simulink model "Lcontainer_simNN"  (R2018b)
settings: Solver=FixedStepAuto  StartTime=0.0  StopTime=50  FixedStep=0.1  RelTol=1e-3
libraries: neural x548, simulink x2
(part 9 of 26)

== system Lcontainer_simNN/Lcontainer Plant/NN Plant LContainer/Layer 5/Delays 1 ==
  "p{5}" : Inport  PortDimensions=30
      mask Display: e = 0.06;c1 = [120 230 180]/255;c2 = ([120 230 180]+0)/(256+128);c3 = ([120 230 180]+128)/(256+128);patch([0 1 1 0],[0 0 1 1],c1);patch([0 1 1 1-e 1-e 0+e],[0 0 1 1-e 0+e 0+e],c2);patch([0 0 1 1-e 0+e 0+e],[0 1 1 1-e 1-e 0+e],c3);plot([0 1 1 0 0],[0 0 1 1 0]);
  mux : Mux  Inputs=1
      mask Display: e = 0.06;c1 = [120 150 230]/255;c2 = ([120 150 230]+0)/383;c3 = ([120 150 230]+128)/383;patch([0 1 1 0],[0 0 1 1],c1);patch([0 1 1 1-e 1-e 0+e],[0 0 1 1-e 0+e 0+e],c2);patch([0 0 1 1-e 0+e 0+e],[0 1 1 1-e 1-e 0+e],c3);plot([0 1 1 0 0],[0 0 1 1 0]);disp('Mux')
  "pd{5,4}" : Outport
      mask Display: e = 0.06;c1 = [120 230 180]/255;c2 = ([120 230 180]+0)/(256+128);c3 = ([120 230 180]+128)/(256+128);patch([0 1 1 0],[0 0 1 1],c1);patch([0 1 1 1-e 1-e 0+e],[0 0 1 1-e 0+e 0+e],c2);patch([0 0 1 1-e 0+e 0+e],[0 1 1 1-e 1-e 0+e],c3);plot([0 1 1 0 0],[0 0 1 1 0]);
  wires:
  mux/1 -> "pd{5,4}"/1
  "p{5}"/1 -> mux/1

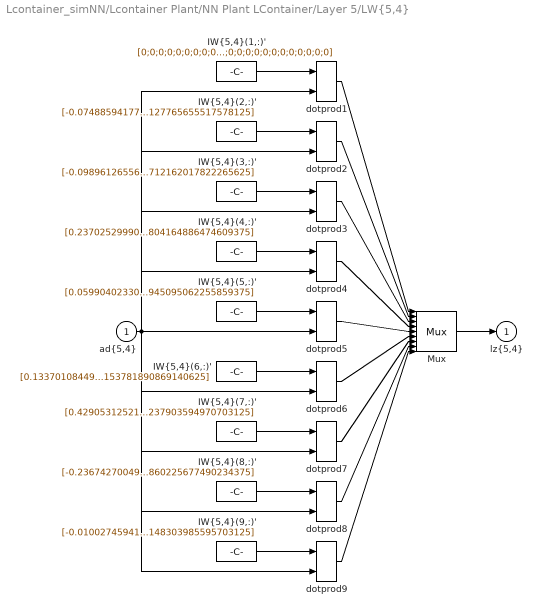
== system Lcontainer_simNN/Lcontainer Plant/NN Plant LContainer/Layer 5/LW{5,4} ==
  "ad{5,4}" : Inport  PortDimensions=30
      mask Display: e = 0.06;c1 = [120 230 180]/255;c2 = ([120 230 180]+0)/(256+128);c3 = ([120 230 180]+128)/(256+128);patch([0 1 1 0],[0 0 1 1],c1);patch([0 1 1 1-e 1-e 0+e],[0 0 1 1-e 0+e 0+e],c2);patch([0 0 1 1-e 0+e 0+e],[0 1 1 1-e 1-e 0+e],c3);plot([0 1 1 0 0],[0 0 1 1 0]);
  "IW{5,4}(1,:)'" : Constant  Value=[0;0;0;0;0;0;0;0;0;0;0;0;0;0;0;0;0;0;0;0;0;0;0;0;0;0;0;0;0;0]
      mask Display: e = 0.06;c1 = [120 150 230]/255;c2 = ([120 150 230]+0)/383;c3 = ([120 150 230]+128)/383;patch([0 1 1 0],[0 0 1 1],c1);patch([0 1 1 1-e 1-e 0+e],[0 0 1 1-e 0+e 0+e],c2);patch([0 0 1 1-e 0+e 0+e],[0 1 1 1-e 1-e 0+e],c3);plot([0 1 1 0 0],[0 0 1 1 0]);disp('weights');
  "IW{5,4}(2,:)'" : Constant  Value=[-0.0748859417790649073420894410446635447442531585693359375;-0.04828556424962082704865906634950079023838043212890625;-0.033114210472323622747037319413720979355275630950927734375;0;-0.1705933706616073741724193268964882008731365203857421875;-0.024529633517243805418406310536738601513206958770751953125;0.0021195137212356375717992040819126486894674599170684814453125;0.01236919402911206000705846008713706396520137786865234375;0;0.14372941073911327247714098120923154056072235107421875;-0.08898138145787300168354505558454548008739948272705078125;0.25399576565349579748698261028039269149303436279296875;0;0;0.0852243252470792078678840653083170764148235321044921875;-0.01075542795457371143819091940940779750235378742218017578125;-0.445323566962354366882692602302995510399341583251953125;0;0;-0.09295428806737338067733844582107849419116973876953125;0;0.01344213504127246376629312152317652362398803234100341796875;0.032260333898478661673880907301281695254147052764892578125;0;0.09247761640926364934411907370304106734693050384521484375;0;-0.168932518774683571027850348400534130632877349853515625;0.0852925813085265438484583455647225491702556610107421875;0;0.06589481023012284943707328466189210303127765655517578125]
      mask Display: e = 0.06;c1 = [120 150 230]/255;c2 = ([120 150 230]+0)/383;c3 = ([120 150 230]+128)/383;patch([0 1 1 0],[0 0 1 1],c1);patch([0 1 1 1-e 1-e 0+e],[0 0 1 1-e 0+e 0+e],c2);patch([0 0 1 1-e 0+e 0+e],[0 1 1 1-e 1-e 0+e],c3);plot([0 1 1 0 0],[0 0 1 1 0]);disp('weights');
  "IW{5,4}(3,:)'" : Constant  Value=[-0.09896126556202029800335395748334121890366077423095703125;0.0796723090629556096597951864168862812221050262451171875;-0.0127063350048920893631265727208301541395485401153564453125;0;0.057556295472263131751677889269558363594114780426025390625;0.2154824786930362723325060869683511555194854736328125;0.000775384221512636306015975318217670064768753945827484130859375;0.0271174472186132727025142941101876203902065753936767578125;0;-0.371698716803673889774728422707994468510150909423828125;-0.146328714086319866538588030380196869373321533203125;0.0713073127667704642629331601710873655974864959716796875;0;0;-0.2355891362308875913722516770576476119458675384521484375;-0.30076611836778355257848716064472682774066925048828125;-0.1185366313755974732035980423461296595633029937744140625;0;0;0.1996103508031047690796100368970655836164951324462890625;0;0.05914976055061747783891945573486736975610256195068359375;0.0178303994357455440622484132973113446496427059173583984375;0;0.1153034810071617843885150023197638802230358123779296875;0;-0.045867220948066007857324422047895495779812335968017578125;0.259149319149599433043107410412630997598171234130859375;0;0.03300873027772155410275445319712162017822265625]
      mask Display: e = 0.06;c1 = [120 150 230]/255;c2 = ([120 150 230]+0)/383;c3 = ([120 150 230]+128)/383;patch([0 1 1 0],[0 0 1 1],c1);patch([0 1 1 1-e 1-e 0+e],[0 0 1 1-e 0+e 0+e],c2);patch([0 0 1 1-e 0+e 0+e],[0 1 1 1-e 1-e 0+e],c3);plot([0 1 1 0 0],[0 0 1 1 0]);disp('weights');
  "IW{5,4}(4,:)'" : Constant  Value=[0.237025299903385555655432881394517607986927032470703125;-0.09628402043828758471999407220209832303225994110107421875;0.1610493651533241032947074700132361613214015960693359375;0;0.1525638746941407053459016651686397381126880645751953125;-0.369699757752953439560172910205437801778316497802734375;0.04575628933936337627841339781298302114009857177734375;-0.0272463917095127523826381121807571616955101490020751953125;0;0.1707957341201938039620955578357097692787647247314453125;0.1980833692316685823442412583972327411174774169921875;0.34262854725739433359166241643833927810192108154296875;0;0;-0.440432226404521121043700304653611965477466583251953125;-0.0306731198290640764969605669421071070246398448944091796875;-0.11361114234840441472584871007711626589298248291015625;0;0;0.161134980998437982169235738183488138020038604736328125;0;-0.1919326921231571392301162859439500607550144195556640625;-0.18954446100379473971742072535562328994274139404296875;0;0.10598471434648359945640549995005130767822265625;0;0.09503752363470081843122017062341910786926746368408203125;0.1143533842217742402258551237537176348268985748291015625;0;-0.6652481266117751257382906260318122804164886474609375]
      mask Display: e = 0.06;c1 = [120 150 230]/255;c2 = ([120 150 230]+0)/383;c3 = ([120 150 230]+128)/383;patch([0 1 1 0],[0 0 1 1],c1);patch([0 1 1 1-e 1-e 0+e],[0 0 1 1-e 0+e 0+e],c2);patch([0 0 1 1-e 0+e 0+e],[0 1 1 1-e 1-e 0+e],c3);plot([0 1 1 0 0],[0 0 1 1 0]);disp('weights');
  "IW{5,4}(5,:)'" : Constant  Value=[0.05990402330856892110233502535265870392322540283203125;0.00141316250715774042491512663133335081511177122592926025390625;-0.2434454959196580003943921610698453150689601898193359375;0;0.0717643993970850380126336176545009948313236236572265625;0.028162462427314925716981264258720329962670803070068359375;0.0094946210627239562007684270383833791129291057586669921875;-0.055190171920815551953598543377665919251739978790283203125;0;-0.0250218219302644727386475409502963884733617305755615234375;0.012124972570229854140766434511533589102327823638916015625;0.13711765032037870337688900690409354865550994873046875;0;0;0.09628367634003372199646975104769808240234851837158203125;-0.00681706128747262829481456947178230620920658111572265625;0.1430879199190295825161456377827562391757965087890625;0;0;0.0239743569962188492195043210131188970990478992462158203125;0;-0.08149740200468764961261314283547108061611652374267578125;0.010347551788515589599182220581496949307620525360107421875;0;0.05234499219716891305065331607693224214017391204833984375;0;0.0880266504674781236072789170066243968904018402099609375;-0.00576249198361480398367096000811216072179377079010009765625;0;0.056000545253366527942429087261189124546945095062255859375]
      mask Display: e = 0.06;c1 = [120 150 230]/255;c2 = ([120 150 230]+0)/383;c3 = ([120 150 230]+128)/383;patch([0 1 1 0],[0 0 1 1],c1);patch([0 1 1 1-e 1-e 0+e],[0 0 1 1-e 0+e 0+e],c2);patch([0 0 1 1-e 0+e 0+e],[0 1 1 1-e 1-e 0+e],c3);plot([0 1 1 0 0],[0 0 1 1 0]);disp('weights');
  "IW{5,4}(6,:)'" : Constant  Value=[0.133701084498613287365742507972754538059234619140625;-0.08509330829521111194679861000622622668743133544921875;-0.0205939214417339526430605900486625614576041698455810546875;0;0.17660601722820679082559536254848353564739227294921875;-0.0985909020102693489651102254356374032795429229736328125;-0.006612346173665164562882612386829350725747644901275634765625;0.035407645810061887103881161920071463100612163543701171875;0;0.12139874970078590177280375428381375968456268310546875;-0.04879072530735041601790413778871879912912845611572265625;0.046767611231733612064953575782055850140750408172607421875;0;0;0.07297241468848725265416987895150668919086456298828125;0.029678867821005351645968772800188162364065647125244140625;0.11596813525751230311566786213006707839667797088623046875;0;0;0.029034809825560538298905299825491965748369693756103515625;0;0.07527837444470493466486260558667709119617938995361328125;-0.02440627391344178664933650679813581518828868865966796875;0;0.138042976115350046750762658120947889983654022216796875;0;-0.07122006785791994143419714191622915677726268768310546875;-0.1535383105928499192227576486402540467679500579833984375;0;0.07388509161200375319200617241222062148153781890869140625]
      mask Display: e = 0.06;c1 = [120 150 230]/255;c2 = ([120 150 230]+0)/383;c3 = ([120 150 230]+128)/383;patch([0 1 1 0],[0 0 1 1],c1);patch([0 1 1 1-e 1-e 0+e],[0 0 1 1-e 0+e 0+e],c2);patch([0 0 1 1-e 0+e 0+e],[0 1 1 1-e 1-e 0+e],c3);plot([0 1 1 0 0],[0 0 1 1 0]);disp('weights');
  "IW{5,4}(7,:)'" : Constant  Value=[0.42905312521970484507249921080074273049831390380859375;0.1906589972924225551142995982445427216589450836181640625;-0.2203038801554847714303519978784606792032718658447265625;0;0.0217157024741243230570031386150731123052537441253662109375;0.00986713763709344722496741297845801454968750476837158203125;-0.0015074870746090672513073371874270378611981868743896484375;-0.00103538587713326683814596407273711520247161388397216796875;0;-0.334719609204135737368090985910384915769100189208984375;-0.321965949665375450461368700416642241179943084716796875;0.030844820817152888980938740814963239245116710662841796875;0;0;0.01779259507096221659683266125284717418253421783447265625;0.3773025667999700960564268825692124664783477783203125;-0.12169499692181691419268219078730908222496509552001953125;0;0;-0.352967196418212225683674887477536685764789581298828125;0;0.37503733804256977890645430306904017925262451171875;-0.0031221649642524753644201584990014453069306910037994384765625;0;-0.12199386878124203470452613373709027655422687530517578125;0;-0.0686099962025387422048794405782246030867099761962890625;0.2458374314142147409878447206210694275796413421630859375;0;-0.262765638305728910228964423367870040237903594970703125]
      mask Display: e = 0.06;c1 = [120 150 230]/255;c2 = ([120 150 230]+0)/383;c3 = ([120 150 230]+128)/383;patch([0 1 1 0],[0 0 1 1],c1);patch([0 1 1 1-e 1-e 0+e],[0 0 1 1-e 0+e 0+e],c2);patch([0 0 1 1-e 0+e 0+e],[0 1 1 1-e 1-e 0+e],c3);plot([0 1 1 0 0],[0 0 1 1 0]);disp('weights');
  "IW{5,4}(8,:)'" : Constant  Value=[-0.23674270049570278473538564867340028285980224609375;-0.036559030986588435252482298665199778042733669281005859375;-0.2257526060123458411244001808881876058876514434814453125;0;0.21935645089634048243709685266367159783840179443359375;0.10110863562139782434456947157741524279117584228515625;-0.0015212242213593590682563228000390154193155467510223388671875;0.01019800474396239352292692359469583607278764247894287109375;0;0.1479307078988518764361970170284621417522430419921875;0.14256822808086611065192528258194215595722198486328125;0.03784177868002285005655238592225941829383373260498046875;0;0;-0.141814798576826162079811410876573063433170318603515625;-0.02754221019145429438790273479753523133695125579833984375;0.275417755016419241176350851674214936792850494384765625;0;0;-0.16649009753270493927601592076825909316539764404296875;0;0.27531561729428222218274413535255007445812225341796875;0.046655242645399143397444419179009855724871158599853515625;0;0.1341753073127237294581703963558538816869258880615234375;0;-0.0941217711476544371951291623190627433359622955322265625;-0.00110793594252062426071259171322935799253173172473907470703125;0;-0.11447492526362222642344335099551244638860225677490234375]
      mask Display: e = 0.06;c1 = [120 150 230]/255;c2 = ([120 150 230]+0)/383;c3 = ([120 150 230]+128)/383;patch([0 1 1 0],[0 0 1 1],c1);patch([0 1 1 1-e 1-e 0+e],[0 0 1 1-e 0+e 0+e],c2);patch([0 0 1 1-e 0+e 0+e],[0 1 1 1-e 1-e 0+e],c3);plot([0 1 1 0 0],[0 0 1 1 0]);disp('weights');
  "IW{5,4}(9,:)'" : Constant  Value=[-0.01002745941681644492593505901822936721146106719970703125;0.0167845265205452676138264678229461424052715301513671875;0.049490530702450581668205842333918553777039051055908203125;0;-0.0284552194108398000260695681618017260916531085968017578125;0.02483904552978373481142426726364647038280963897705078125;0.00189694606096295803783491340510636291583068668842315673828125;0.0047821216244630405933779826455065631307661533355712890625;0;-0.0285485124585271067554348434214261942543089389801025390625;-0.02441746492862141570956424629912362433969974517822265625;0.005519148991629414628679040077940953779034316539764404296875;0;0;-0.0242204291869716932528167063765067723579704761505126953125;-0.062014224507974675948407394798778113909065723419189453125;-0.09427889191645007216369123170807142741978168487548828125;0;0;0.04528510720060403837994300602076691575348377227783203125;0;-0.010634689821550184773979452756975661031901836395263671875;-0.0113809821653901577231948749613366089761257171630859375;0;0.01434108884514245611796479096256007323972880840301513671875;0;-0.006045715600746133511211866107259993441402912139892578125;0.10052070987340717966862513321757433004677295684814453125;0;0.0453833762214126690270887820588541217148303985595703125]
      mask Display: e = 0.06;c1 = [120 150 230]/255;c2 = ([120 150 230]+0)/383;c3 = ([120 150 230]+128)/383;patch([0 1 1 0],[0 0 1 1],c1);patch([0 1 1 1-e 1-e 0+e],[0 0 1 1-e 0+e 0+e],c2);patch([0 0 1 1-e 0+e 0+e],[0 1 1 1-e 1-e 0+e],c3);plot([0 1 1 0 0],[0 0 1 1 0]);disp('weights');
  Mux : Mux  Inputs=9
      mask Display: e = 0.06;c1 = [120 150 230]/255;c2 = ([120 150 230]+0)/383;c3 = ([120 150 230]+128)/383;patch([0 1 1 0],[0 0 1 1],c1);patch([0 1 1 1-e 1-e 0+e],[0 0 1 1-e 0+e 0+e],c2);patch([0 0 1 1-e 0+e 0+e],[0 1 1 1-e 1-e 0+e],c3);plot([0 1 1 0 0],[0 0 1 1 0]);disp('Mux');
  dotprod{1..9} (9 alike) : neural/Weight Functions/dotprod
  "lz{5,4}" : Outport
      mask Display: e = 0.06;c1 = [120 230 180]/255;c2 = ([120 230 180]+0)/(256+128);c3 = ([120 230 180]+128)/(256+128);patch([0 1 1 0],[0 0 1 1],c1);patch([0 1 1 1-e 1-e 0+e],[0 0 1 1-e 0+e 0+e],c2);patch([0 0 1 1-e 0+e 0+e],[0 1 1 1-e 1-e 0+e],c3);plot([0 1 1 0 0],[0 0 1 1 0]);
  wires:
  Mux/1 -> "lz{5,4}"/1
  dotprod9/1 -> Mux/9
  "IW{5,4}(9,:)'"/1 -> dotprod9/1
  dotprod8/1 -> Mux/8
  "IW{5,4}(8,:)'"/1 -> dotprod8/1
  dotprod7/1 -> Mux/7
  "IW{5,4}(7,:)'"/1 -> dotprod7/1
  dotprod6/1 -> Mux/6
  "IW{5,4}(6,:)'"/1 -> dotprod6/1
  dotprod5/1 -> Mux/5
  "IW{5,4}(5,:)'"/1 -> dotprod5/1
  dotprod4/1 -> Mux/4
  "IW{5,4}(4,:)'"/1 -> dotprod4/1
  dotprod3/1 -> Mux/3
  "IW{5,4}(3,:)'"/1 -> dotprod3/1
  dotprod2/1 -> Mux/2
  "IW{5,4}(2,:)'"/1 -> dotprod2/1
  dotprod1/1 -> Mux/1
  "ad{5,4}"/1 -> dotprod9/2, dotprod8/2, dotprod7/2, dotprod6/2, dotprod5/2, dotprod4/2, dotprod3/2, dotprod2/2, dotprod1/2
  "IW{5,4}(1,:)'"/1 -> dotprod1/1

== system Lcontainer_simNN/Lcontainer Plant/NN Plant2 LContainer /Layer 1/Delays 1 ==
  "p{1}" : Inport  PortDimensions=10
      mask Display: e = 0.06;c1 = [120 230 180]/255;c2 = ([120 230 180]+0)/(256+128);c3 = ([120 230 180]+128)/(256+128);patch([0 1 1 0],[0 0 1 1],c1);patch([0 1 1 1-e 1-e 0+e],[0 0 1 1-e 0+e 0+e],c2);patch([0 0 1 1-e 0+e 0+e],[0 1 1 1-e 1-e 0+e],c3);plot([0 1 1 0 0],[0 0 1 1 0]);
  mux : Mux  Inputs=1
      mask Display: e = 0.06;c1 = [120 150 230]/255;c2 = ([120 150 230]+0)/383;c3 = ([120 150 230]+128)/383;patch([0 1 1 0],[0 0 1 1],c1);patch([0 1 1 1-e 1-e 0+e],[0 0 1 1-e 0+e 0+e],c2);patch([0 0 1 1-e 0+e 0+e],[0 1 1 1-e 1-e 0+e],c3);plot([0 1 1 0 0],[0 0 1 1 0]);disp('Mux')
  "pd{1,1}" : Outport
      mask Display: e = 0.06;c1 = [120 230 180]/255;c2 = ([120 230 180]+0)/(256+128);c3 = ([120 230 180]+128)/(256+128);patch([0 1 1 0],[0 0 1 1],c1);patch([0 1 1 1-e 1-e 0+e],[0 0 1 1-e 0+e 0+e],c2);patch([0 0 1 1-e 0+e 0+e],[0 1 1 1-e 1-e 0+e],c3);plot([0 1 1 0 0],[0 0 1 1 0]);
  wires:
  mux/1 -> "pd{1,1}"/1
  "p{1}"/1 -> mux/1
